simulink library "STMM"  (R2024a)
settings: Solver=VariableStepAuto  StartTime=0.0  StopTime=10.0  RelTol=1e-3
undefined symbols (not defined in the file or in its folder): raptor_xcp_function, StateCAN
libraries: Utilities x260, Raptor_lib x68, simulink x2
(part 2 of 3)

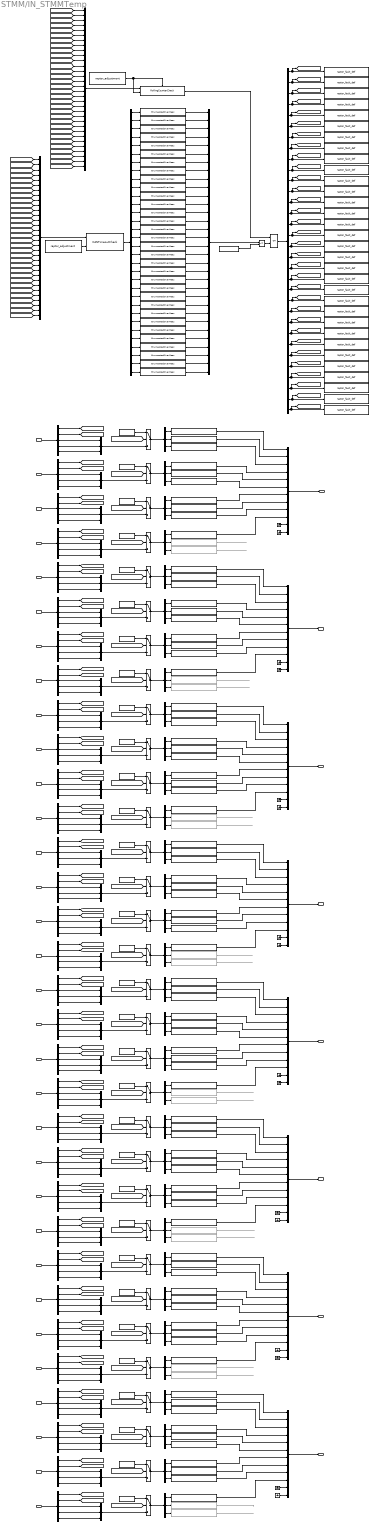
== system STMM/IN_STMMTemp ==
  IO_CAN2_300_Bus : Inport
  IO_CAN2_301_Bus : Inport  Port=2
  IO_CAN2_302_Bus : Inport  Port=3
  IO_CAN2_303_Bus : Inport  Port=4
  IO_CAN2_304_Bus : Inport  Port=5
  IO_CAN2_305_Bus : Inport  Port=6
  IO_CAN2_306_Bus : Inport  Port=7
  IO_CAN2_307_Bus : Inport  Port=8
  IO_CAN2_308_Bus : Inport  Port=9
  IO_CAN2_309_Bus : Inport  Port=10
  IO_CAN2_310_Bus : Inport  Port=11
  IO_CAN2_311_Bus : Inport  Port=12
  IO_CAN2_312_Bus : Inport  Port=13
  IO_CAN2_313_Bus : Inport  Port=14
  IO_CAN2_314_Bus : Inport  Port=15
  IO_CAN2_315_Bus : Inport  Port=16
  IO_CAN2_316_Bus : Inport  Port=17
  IO_CAN2_317_Bus : Inport  Port=18
  IO_CAN2_318_Bus : Inport  Port=19
  IO_CAN2_319_Bus : Inport  Port=20
  IO_CAN2_320_Bus : Inport  Port=21
  IO_CAN2_321_Bus : Inport  Port=22
  IO_CAN2_322_Bus : Inport  Port=23
  IO_CAN2_323_Bus : Inport  Port=24
  IO_CAN2_324_Bus : Inport  Port=25
  IO_CAN2_325_Bus : Inport  Port=26
  IO_CAN2_326_Bus : Inport  Port=27
  IO_CAN2_327_Bus : Inport  Port=28
  IO_CAN2_328_Bus : Inport  Port=29
  IO_CAN2_329_Bus : Inport  Port=30
  IO_CAN2_330_Bus : Inport  Port=31
  IO_CAN2_331_Bus : Inport  Port=32
  Bus Creator{,1..7} (8 alike) : BusCreator  Inputs=12
  Bus Selector : BusSelector  OutputSignals=Age,STMM_counterMsg300,STMM_segmentTemp100,STMM_segmentTemp101,STMM_segmentTemp102
  Bus Selector1 : BusSelector  OutputSignals=Age,STMM_counterMsg301,STMM_segmentTemp103,STMM_segmentTemp104,STMM_segmentTemp105
  Bus Selector10 : BusSelector  OutputSignals=Age,STMM_counterMsg310,STMM_segmentTemp306,STMM_segmentTemp307,STMM_segmentTemp308
  Bus Selector11 : BusSelector  OutputSignals=Age,STMM_counterMsg311,STMM_segmentTemp309,STMM_segmentTemp310,STMM_segmentTemp311
  Bus Selector12 : BusSelector  OutputSignals=Age,STMM_counterMsg312,STMM_segmentTemp400,STMM_segmentTemp401,STMM_segmentTemp402
  Bus Selector13 : BusSelector  OutputSignals=Age,STMM_counterMsg313,STMM_segmentTemp403,STMM_segmentTemp404,STMM_segmentTemp405
  Bus Selector14 : BusSelector  OutputSignals=Age,STMM_counterMsg314,STMM_segmentTemp406,STMM_segmentTemp407,STMM_segmentTemp408
  Bus Selector15 : BusSelector  OutputSignals=Age,STMM_counterMsg315,STMM_segmentTemp409,STMM_segmentTemp410,STMM_segmentTemp411
  Bus Selector16 : BusSelector  OutputSignals=Age,STMM_counterMsg316,STMM_segmentTemp500,STMM_segmentTemp501,STMM_segmentTemp502
  Bus Selector17 : BusSelector  OutputSignals=Age,STMM_counterMsg317,STMM_segmentTemp503,STMM_segmentTemp504,STMM_segmentTemp505
  Bus Selector18 : BusSelector  OutputSignals=Age,STMM_counterMsg318,STMM_segmentTemp506,STMM_segmentTemp507,STMM_segmentTemp508
  Bus Selector19 : BusSelector  OutputSignals=Age,STMM_counterMsg319,STMM_segmentTemp509,STMM_segmentTemp510,STMM_segmentTemp511
  Bus Selector2 : BusSelector  OutputSignals=Age,STMM_counterMsg302,STMM_segmentTemp106,STMM_segmentTemp107,STMM_segmentTemp108
  Bus Selector20 : BusSelector  OutputSignals=Age,STMM_counterMsg320,STMM_segmentTemp600,STMM_segmentTemp601,STMM_segmentTemp602
  Bus Selector21 : BusSelector  OutputSignals=Age,STMM_counterMsg321,STMM_segmentTemp603,STMM_segmentTemp604,STMM_segmentTemp605
  Bus Selector22 : BusSelector  OutputSignals=Age,STMM_counterMsg322,STMM_segmentTemp606,STMM_segmentTemp607,STMM_segmentTemp608
  Bus Selector23 : BusSelector  OutputSignals=Age,STMM_counterMsg323,STMM_segmentTemp609,STMM_segmentTemp610,STMM_segmentTemp611
  Bus Selector24 : BusSelector  OutputSignals=Age,STMM_counterMsg324,STMM_segmentTemp700,STMM_segmentTemp701,STMM_segmentTemp702
  Bus Selector25 : BusSelector  OutputSignals=Age,STMM_counterMsg325,STMM_segmentTemp703,STMM_segmentTemp704,STMM_segmentTemp705
  Bus Selector26 : BusSelector  OutputSignals=Age,STMM_counterMsg326,STMM_segmentTemp706,STMM_segmentTemp707,STMM_segmentTemp708
  Bus Selector27 : BusSelector  OutputSignals=Age,STMM_counterMsg327,STMM_segmentTemp709,STMM_segmentTemp710,STMM_segmentTemp711
  Bus Selector28 : BusSelector  OutputSignals=Age,STMM_counterMsg328,STMM_segmentTemp800,STMM_segmentTemp801,STMM_segmentTemp802
  Bus Selector29 : BusSelector  OutputSignals=Age,STMM_counterMsg329,STMM_segmentTemp803,STMM_segmentTemp804,STMM_segmentTemp805
  Bus Selector3 : BusSelector  OutputSignals=Age,STMM_counterMsg303,STMM_segmentTemp109,STMM_segmentTemp110,STMM_segmentTemp111
  Bus Selector30 : BusSelector  OutputSignals=Age,STMM_counterMsg330,STMM_segmentTemp806,STMM_segmentTemp807,STMM_segmentTemp808
  Bus Selector31 : BusSelector  OutputSignals=Age,STMM_counterMsg331,STMM_segmentTemp809,STMM_segmentTemp810,STMM_segmentTemp811
  Bus Selector4 : BusSelector  OutputSignals=Age,STMM_counterMsg304,STMM_segmentTemp200,STMM_segmentTemp201,STMM_segmentTemp202
  Bus Selector5 : BusSelector  OutputSignals=Age,STMM_counterMsg305,STMM_segmentTemp203,STMM_segmentTemp204,STMM_segmentTemp205
  Bus Selector6 : BusSelector  OutputSignals=Age,STMM_counterMsg306,STMM_segmentTemp206,STMM_segmentTemp207,STMM_segmentTemp208
  Bus Selector7 : BusSelector  OutputSignals=Age,STMM_counterMsg307,STMM_segmentTemp209,STMM_segmentTemp210,STMM_segmentTemp211
  Bus Selector8 : BusSelector  OutputSignals=Age,STMM_counterMsg308,STMM_segmentTemp300,STMM_segmentTemp301,STMM_segmentTemp302
  Bus Selector9 : BusSelector  OutputSignals=Age,STMM_counterMsg309,STMM_segmentTemp303,STMM_segmentTemp304,STMM_segmentTemp305
  CANTimeoutCheck : Utilities/CANTimeoutCheck
  Constant{1..32} (32 alike) : Constant  Value=int16(32767)
  Demux : Demux  Outputs=32
  Demux1 : Demux  Outputs=32
  Demux{2..33} (32 alike) : Demux  Outputs=3
  Enumerated Constant : simulink/Sources/Enumerated Constant  OutDataTypeStr=Enum: StateCAN  Value=StateCAN.Normal  SampleTime=inf
  EnumeratedOverMeas1 : Utilities/EnumeratedOverMeas  sigName='IN_CAN2_300_Status_en'  enumName='StateCAN'
  EnumeratedOverMeas10 : Utilities/EnumeratedOverMeas  sigName='IN_CAN2_309_Status_en'  enumName='StateCAN'
  EnumeratedOverMeas11 : Utilities/EnumeratedOverMeas  sigName='IN_CAN2_310_Status_en'  enumName='StateCAN'
  EnumeratedOverMeas12 : Utilities/EnumeratedOverMeas  sigName='IN_CAN2_311_Status_en'  enumName='StateCAN'
  EnumeratedOverMeas13 : Utilities/EnumeratedOverMeas  sigName='IN_CAN2_312_Status_en'  enumName='StateCAN'
  EnumeratedOverMeas14 : Utilities/EnumeratedOverMeas  sigName='IN_CAN2_313_Status_en'  enumName='StateCAN'
  EnumeratedOverMeas15 : Utilities/EnumeratedOverMeas  sigName='IN_CAN2_314_Status_en'  enumName='StateCAN'
  EnumeratedOverMeas16 : Utilities/EnumeratedOverMeas  sigName='IN_CAN2_315_Status_en'  enumName='StateCAN'
  EnumeratedOverMeas17 : Utilities/EnumeratedOverMeas  sigName='IN_CAN2_316_Status_en'  enumName='StateCAN'
  EnumeratedOverMeas18 : Utilities/EnumeratedOverMeas  sigName='IN_CAN2_317_Status_en'  enumName='StateCAN'
  EnumeratedOverMeas19 : Utilities/EnumeratedOverMeas  sigName='IN_CAN2_318_Status_en'  enumName='StateCAN'
  EnumeratedOverMeas2 : Utilities/EnumeratedOverMeas  sigName='IN_CAN2_301_Status_en'  enumName='StateCAN'
  EnumeratedOverMeas20 : Utilities/EnumeratedOverMeas  sigName='IN_CAN2_319_Status_en'  enumName='StateCAN'
  EnumeratedOverMeas21 : Utilities/EnumeratedOverMeas  sigName='IN_CAN2_320_Status_en'  enumName='StateCAN'
  EnumeratedOverMeas22 : Utilities/EnumeratedOverMeas  sigName='IN_CAN2_321_Status_en'  enumName='StateCAN'
  EnumeratedOverMeas23 : Utilities/EnumeratedOverMeas  sigName='IN_CAN2_322_Status_en'  enumName='StateCAN'
  EnumeratedOverMeas24 : Utilities/EnumeratedOverMeas  sigName='IN_CAN2_323_Status_en'  enumName='StateCAN'
  EnumeratedOverMeas25 : Utilities/EnumeratedOverMeas  sigName='IN_CAN2_324_Status_en'  enumName='StateCAN'
  EnumeratedOverMeas26 : Utilities/EnumeratedOverMeas  sigName='IN_CAN2_325_Status_en'  enumName='StateCAN'
  EnumeratedOverMeas27 : Utilities/EnumeratedOverMeas  sigName='IN_CAN2_326_Status_en'  enumName='StateCAN'
  EnumeratedOverMeas28 : Utilities/EnumeratedOverMeas  sigName='IN_CAN2_327_Status_en'  enumName='StateCAN'
  EnumeratedOverMeas29 : Utilities/EnumeratedOverMeas  sigName='IN_CAN2_328_Status_en'  enumName='StateCAN'
  EnumeratedOverMeas3 : Utilities/EnumeratedOverMeas  sigName='IN_CAN2_302_Status_en'  enumName='StateCAN'
  EnumeratedOverMeas30 : Utilities/EnumeratedOverMeas  sigName='IN_CAN2_329_Status_en'  enumName='StateCAN'
  EnumeratedOverMeas31 : Utilities/EnumeratedOverMeas  sigName='IN_CAN2_330_Status_en'  enumName='StateCAN'
  EnumeratedOverMeas32 : Utilities/EnumeratedOverMeas  sigName='IN_CAN2_331_Status_en'  enumName='StateCAN'
  EnumeratedOverMeas4 : Utilities/EnumeratedOverMeas  sigName='IN_CAN2_303_Status_en'  enumName='StateCAN'
  EnumeratedOverMeas5 : Utilities/EnumeratedOverMeas  sigName='IN_CAN2_304_Status_en'  enumName='StateCAN'
  EnumeratedOverMeas6 : Utilities/EnumeratedOverMeas  sigName='IN_CAN2_305_Status_en'  enumName='StateCAN'
  EnumeratedOverMeas7 : Utilities/EnumeratedOverMeas  sigName='IN_CAN2_306_Status_en'  enumName='StateCAN'
  EnumeratedOverMeas8 : Utilities/EnumeratedOverMeas  sigName='IN_CAN2_307_Status_en'  enumName='StateCAN'
  EnumeratedOverMeas9 : Utilities/EnumeratedOverMeas  sigName='IN_CAN2_308_Status_en'  enumName='StateCAN'
  Equal : RelationalOperator  Operator=~=  OutDataTypeStr=boolean  RndMeth=Simplest  InputSameDT=off
  Ground{,1..15} (16 alike) : Ground
  Mux{,1..31} (32 alike) : Mux  Inputs=3
  Mux32 : Mux  Inputs=32
  Mux33 : Mux  Inputs=32
  Mux34 : Mux  Inputs=32
  OR : Logic  Operator=OR  AllPortsSameDT=off  OutDataTypeStr=boolean
  OverMeas : Utilities/OverMeas  sigName='IN_SegmentTemp100_degC'  minimum=-inf  maximum=inf
  OverMeas1 : Utilities/OverMeas  sigName='IN_SegmentTemp101_degC'  minimum=-inf  maximum=inf
  OverMeas10 : Utilities/OverMeas  Commented=on  sigName='IN_SegmentTemp110_degC'  minimum=-inf  maximum=inf
  OverMeas11 : Utilities/OverMeas  Commented=on  sigName='IN_SegmentTemp111_degC'  minimum=-inf  maximum=inf
  OverMeas12 : Utilities/OverMeas  sigName='IN_SegmentTemp200_degC'  minimum=-inf  maximum=inf
  OverMeas13 : Utilities/OverMeas  sigName='IN_SegmentTemp201_degC'  minimum=-inf  maximum=inf
  OverMeas14 : Utilities/OverMeas  Commented=on  sigName='IN_SegmentTemp210_degC'  minimum=-inf  maximum=inf
  OverMeas15 : Utilities/OverMeas  Commented=on  sigName='IN_SegmentTemp211_degC'  minimum=-inf  maximum=inf
  OverMeas16 : Utilities/OverMeas  sigName='IN_SegmentTemp202_degC'  minimum=-inf  maximum=inf
  OverMeas17 : Utilities/OverMeas  sigName='IN_SegmentTemp203_degC'  minimum=-inf  maximum=inf
  OverMeas18 : Utilities/OverMeas  sigName='IN_SegmentTemp204_degC'  minimum=-inf  maximum=inf
  OverMeas19 : Utilities/OverMeas  sigName='IN_SegmentTemp205_degC'  minimum=-inf  maximum=inf
  OverMeas2 : Utilities/OverMeas  sigName='IN_SegmentTemp102_degC'  minimum=-inf  maximum=inf
  OverMeas20 : Utilities/OverMeas  sigName='IN_SegmentTemp206_degC'  minimum=-inf  maximum=inf
  OverMeas21 : Utilities/OverMeas  sigName='IN_SegmentTemp207_degC'  minimum=-inf  maximum=inf
  OverMeas22 : Utilities/OverMeas  sigName='IN_SegmentTemp208_degC'  minimum=-inf  maximum=inf
  OverMeas23 : Utilities/OverMeas  sigName='IN_SegmentTemp209_degC'  minimum=-inf  maximum=inf
  OverMeas24 : Utilities/OverMeas  sigName='IN_SegmentTemp300_degC'  minimum=-inf  maximum=inf
  OverMeas25 : Utilities/OverMeas  sigName='IN_SegmentTemp301_degC'  minimum=-inf  maximum=inf
  OverMeas26 : Utilities/OverMeas  Commented=on  sigName='IN_SegmentTemp310_degC'  minimum=-inf  maximum=inf
  OverMeas27 : Utilities/OverMeas  Commented=on  sigName='IN_SegmentTemp311_degC'  minimum=-inf  maximum=inf
  OverMeas28 : Utilities/OverMeas  sigName='IN_SegmentTemp302_degC'  minimum=-inf  maximum=inf
  OverMeas29 : Utilities/OverMeas  sigName='IN_SegmentTemp303_degC'  minimum=-inf  maximum=inf
  OverMeas3 : Utilities/OverMeas  sigName='IN_SegmentTemp103_degC'  minimum=-inf  maximum=inf
  OverMeas30 : Utilities/OverMeas  sigName='IN_SegmentTemp304_degC'  minimum=-inf  maximum=inf
  OverMeas31 : Utilities/OverMeas  sigName='IN_SegmentTemp305_degC'  minimum=-inf  maximum=inf
  OverMeas32 : Utilities/OverMeas  sigName='IN_SegmentTemp306_degC'  minimum=-inf  maximum=inf
  OverMeas33 : Utilities/OverMeas  sigName='IN_SegmentTemp307_degC'  minimum=-inf  maximum=inf
  OverMeas34 : Utilities/OverMeas  sigName='IN_SegmentTemp308_degC'  minimum=-inf  maximum=inf
  OverMeas35 : Utilities/OverMeas  sigName='IN_SegmentTemp309_degC'  minimum=-inf  maximum=inf
  OverMeas36 : Utilities/OverMeas  sigName='IN_SegmentTemp400_degC'  minimum=-inf  maximum=inf
  OverMeas37 : Utilities/OverMeas  sigName='IN_SegmentTemp401_degC'  minimum=-inf  maximum=inf
  OverMeas38 : Utilities/OverMeas  Commented=on  sigName='IN_SegmentTemp410_degC'  minimum=-inf  maximum=inf
  OverMeas39 : Utilities/OverMeas  Commented=on  sigName='IN_SegmentTemp411_degC'  minimum=-inf  maximum=inf
  OverMeas4 : Utilities/OverMeas  sigName='IN_SegmentTemp104_degC'  minimum=-inf  maximum=inf
  OverMeas40 : Utilities/OverMeas  sigName='IN_SegmentTemp402_degC'  minimum=-inf  maximum=inf
  OverMeas41 : Utilities/OverMeas  sigName='IN_SegmentTemp403_degC'  minimum=-inf  maximum=inf
  OverMeas42 : Utilities/OverMeas  sigName='IN_SegmentTemp404_degC'  minimum=-inf  maximum=inf
  OverMeas43 : Utilities/OverMeas  sigName='IN_SegmentTemp405_degC'  minimum=-inf  maximum=inf
  OverMeas44 : Utilities/OverMeas  sigName='IN_SegmentTemp406_degC'  minimum=-inf  maximum=inf
  OverMeas45 : Utilities/OverMeas  sigName='IN_SegmentTemp407_degC'  minimum=-inf  maximum=inf
  OverMeas46 : Utilities/OverMeas  sigName='IN_SegmentTemp408_degC'  minimum=-inf  maximum=inf
  OverMeas47 : Utilities/OverMeas  sigName='IN_SegmentTemp409_degC'  minimum=-inf  maximum=inf
  OverMeas48 : Utilities/OverMeas  sigName='IN_SegmentTemp500_degC'  minimum=-inf  maximum=inf
  OverMeas49 : Utilities/OverMeas  sigName='IN_SegmentTemp501_degC'  minimum=-inf  maximum=inf
  OverMeas5 : Utilities/OverMeas  sigName='IN_SegmentTemp105_degC'  minimum=-inf  maximum=inf
  OverMeas50 : Utilities/OverMeas  Commented=on  sigName='IN_SegmentTemp510_degC'  minimum=-inf  maximum=inf
  OverMeas51 : Utilities/OverMeas  Commented=on  sigName='IN_SegmentTemp511_degC'  minimum=-inf  maximum=inf
  OverMeas52 : Utilities/OverMeas  sigName='IN_SegmentTemp502_degC'  minimum=-inf  maximum=inf
  OverMeas53 : Utilities/OverMeas  sigName='IN_SegmentTemp503_degC'  minimum=-inf  maximum=inf
  OverMeas54 : Utilities/OverMeas  sigName='IN_SegmentTemp504_degC'  minimum=-inf  maximum=inf
  OverMeas55 : Utilities/OverMeas  sigName='IN_SegmentTemp505_degC'  minimum=-inf  maximum=inf
  OverMeas56 : Utilities/OverMeas  sigName='IN_SegmentTemp506_degC'  minimum=-inf  maximum=inf
  OverMeas57 : Utilities/OverMeas  sigName='IN_SegmentTemp507_degC'  minimum=-inf  maximum=inf
  OverMeas58 : Utilities/OverMeas  sigName='IN_SegmentTemp508_degC'  minimum=-inf  maximum=inf
  OverMeas59 : Utilities/OverMeas  sigName='IN_SegmentTemp509_degC'  minimum=-inf  maximum=inf
  OverMeas6 : Utilities/OverMeas  sigName='IN_SegmentTemp106_degC'  minimum=-inf  maximum=inf
  OverMeas60 : Utilities/OverMeas  sigName='IN_SegmentTemp600_degC'  minimum=-inf  maximum=inf
  OverMeas61 : Utilities/OverMeas  sigName='IN_SegmentTemp601_degC'  minimum=-inf  maximum=inf
  OverMeas62 : Utilities/OverMeas  Commented=on  sigName='IN_SegmentTemp610_degC'  minimum=-inf  maximum=inf
  OverMeas63 : Utilities/OverMeas  Commented=on  sigName='IN_SegmentTemp611_degC'  minimum=-inf  maximum=inf
  OverMeas64 : Utilities/OverMeas  sigName='IN_SegmentTemp602_degC'  minimum=-inf  maximum=inf
  OverMeas65 : Utilities/OverMeas  sigName='IN_SegmentTemp603_degC'  minimum=-inf  maximum=inf
  OverMeas66 : Utilities/OverMeas  sigName='IN_SegmentTemp604_degC'  minimum=-inf  maximum=inf
  OverMeas67 : Utilities/OverMeas  sigName='IN_SegmentTemp605_degC'  minimum=-inf  maximum=inf
  OverMeas68 : Utilities/OverMeas  sigName='IN_SegmentTemp606_degC'  minimum=-inf  maximum=inf
  OverMeas69 : Utilities/OverMeas  sigName='IN_SegmentTemp607_degC'  minimum=-inf  maximum=inf
  OverMeas7 : Utilities/OverMeas  sigName='IN_SegmentTemp107_degC'  minimum=-inf  maximum=inf
  OverMeas70 : Utilities/OverMeas  sigName='IN_SegmentTemp608_degC'  minimum=-inf  maximum=inf
  OverMeas71 : Utilities/OverMeas  sigName='IN_SegmentTemp609_degC'  minimum=-inf  maximum=inf
  OverMeas72 : Utilities/OverMeas  sigName='IN_SegmentTemp700_degC'  minimum=-inf  maximum=inf
  OverMeas73 : Utilities/OverMeas  sigName='IN_SegmentTemp701_degC'  minimum=-inf  maximum=inf
  OverMeas74 : Utilities/OverMeas  Commented=on  sigName='IN_SegmentTemp710_degC'  minimum=-inf  maximum=inf
  OverMeas75 : Utilities/OverMeas  Commented=on  sigName='IN_SegmentTemp711_degC'  minimum=-inf  maximum=inf
  OverMeas76 : Utilities/OverMeas  sigName='IN_SegmentTemp702_degC'  minimum=-inf  maximum=inf
  OverMeas77 : Utilities/OverMeas  sigName='IN_SegmentTemp703_degC'  minimum=-inf  maximum=inf
  OverMeas78 : Utilities/OverMeas  sigName='IN_SegmentTemp704_degC'  minimum=-inf  maximum=inf
  OverMeas79 : Utilities/OverMeas  sigName='IN_SegmentTemp705_degC'  minimum=-inf  maximum=inf
  OverMeas8 : Utilities/OverMeas  sigName='IN_SegmentTemp108_degC'  minimum=-inf  maximum=inf
  OverMeas80 : Utilities/OverMeas  sigName='IN_SegmentTemp706_degC'  minimum=-inf  maximum=inf
  OverMeas81 : Utilities/OverMeas  sigName='IN_SegmentTemp707_degC'  minimum=-inf  maximum=inf
  OverMeas82 : Utilities/OverMeas  sigName='IN_SegmentTemp708_degC'  minimum=-inf  maximum=inf
  OverMeas83 : Utilities/OverMeas  sigName='IN_SegmentTemp709_degC'  minimum=-inf  maximum=inf
  OverMeas84 : Utilities/OverMeas  sigName='IN_SegmentTemp800_degC'  minimum=-inf  maximum=inf
  OverMeas85 : Utilities/OverMeas  sigName='IN_SegmentTemp801_degC'  minimum=-inf  maximum=inf
  OverMeas86 : Utilities/OverMeas  Commented=on  sigName='IN_SegmentTemp810_degC'  minimum=-inf  maximum=inf
  OverMeas87 : Utilities/OverMeas  Commented=on  sigName='IN_SegmentTemp811_degC'  minimum=-inf  maximum=inf
  OverMeas88 : Utilities/OverMeas  sigName='IN_SegmentTemp802_degC'  minimum=-inf  maximum=inf
  OverMeas89 : Utilities/OverMeas  sigName='IN_SegmentTemp803_degC'  minimum=-inf  maximum=inf
  OverMeas9 : Utilities/OverMeas  sigName='IN_SegmentTemp109_degC'  minimum=-inf  maximum=inf
  OverMeas90 : Utilities/OverMeas  sigName='IN_SegmentTemp804_degC'  minimum=-inf  maximum=inf
  OverMeas91 : Utilities/OverMeas  sigName='IN_SegmentTemp805_degC'  minimum=-inf  maximum=inf
  OverMeas92 : Utilities/OverMeas  sigName='IN_SegmentTemp806_degC'  minimum=-inf  maximum=inf
  OverMeas93 : Utilities/OverMeas  sigName='IN_SegmentTemp807_degC'  minimum=-inf  maximum=inf
  OverMeas94 : Utilities/OverMeas  sigName='IN_SegmentTemp808_degC'  minimum=-inf  maximum=inf
  OverMeas95 : Utilities/OverMeas  sigName='IN_SegmentTemp809_degC'  minimum=-inf  maximum=inf
  RollingCounterCheck : Utilities/RollingCounterCheck
  Switch{1..32} (32 alike) : Switch  Criteria=u2 ~= 0  SaturateOnIntegerOverflow=off  InputSameDT=off
  raptor_adjustment : Raptor_lib/Data Storage/raptor_adjustment  paramName='IN_STMMTempTOThresh_na'  nameSource=Parameter  initValue=200  dataType=uint32  storage=Calibration  calDispType=Number  calEnum={'False', 'True'}  calGain=1.0  calOffset=0.0  calMax=inf  calMin=-inf  calFormat='-1'  calUnit=''  calHelp=''  calAccess=1  calFunction=raptor_xcp_function(gcb)  calDispHeaders=off  calColHeaders={'Col1' 'Col2' 'Col3'}  calRowHeaders={'Row1' 'Row2' 'Row3'}
      settings: SourceProductName=Raptor
  raptor_adjustment1 : Raptor_lib/Data Storage/raptor_adjustment  paramName='IN_STMMTempRollingCounterEnable_bool'  nameSource=Parameter  initValue=1  dataType=boolean  storage=Calibration  calDispType=Number  calEnum={'False', 'True'}  calGain=1.0  calOffset=0.0  calMax=inf  calMin=-inf  calFormat='-1'  calUnit=''  calHelp=''  calAccess=1  calFunction=raptor_xcp_function(gcb)  calDispHeaders=off  calColHeaders={'Col1' 'Col2' 'Col3'}  calRowHeaders={'Row1' 'Row2' 'Row3'}
      settings: SourceProductName=Raptor
  raptor_fault_def : Raptor_lib/Faults/raptor_fault_def  faultName='IN_CAN2_300_Fault'  persist=on  sticky=off  emisRelated=off  singleTrip=off  clearMethod=Standard  xLimit=25  yLimit=50  calEnable=on  addDisable=off  calAccess=1  calFunction='System | FaultManager'
      settings: SourceProductName=Raptor
  raptor_fault_def1 : Raptor_lib/Faults/raptor_fault_def  faultName='IN_CAN2_301_Fault'  persist=on  sticky=off  emisRelated=off  singleTrip=off  clearMethod=Standard  xLimit=25  yLimit=50  calEnable=on  addDisable=off  calAccess=1  calFunction='System | FaultManager'
      settings: SourceProductName=Raptor
  raptor_fault_def10 : Raptor_lib/Faults/raptor_fault_def  faultName='IN_CAN2_310_Fault'  persist=on  sticky=off  emisRelated=off  singleTrip=off  clearMethod=Standard  xLimit=25  yLimit=50  calEnable=on  addDisable=off  calAccess=1  calFunction='System | FaultManager'
      settings: SourceProductName=Raptor
  raptor_fault_def11 : Raptor_lib/Faults/raptor_fault_def  faultName='IN_CAN2_311_Fault'  persist=on  sticky=off  emisRelated=off  singleTrip=off  clearMethod=Standard  xLimit=25  yLimit=50  calEnable=on  addDisable=off  calAccess=1  calFunction='System | FaultManager'
      settings: SourceProductName=Raptor
  raptor_fault_def12 : Raptor_lib/Faults/raptor_fault_def  faultName='IN_CAN2_312_Fault'  persist=on  sticky=off  emisRelated=off  singleTrip=off  clearMethod=Standard  xLimit=25  yLimit=50  calEnable=on  addDisable=off  calAccess=1  calFunction='System | FaultManager'
      settings: SourceProductName=Raptor
  raptor_fault_def13 : Raptor_lib/Faults/raptor_fault_def  faultName='IN_CAN2_313_Fault'  persist=on  sticky=off  emisRelated=off  singleTrip=off  clearMethod=Standard  xLimit=25  yLimit=50  calEnable=on  addDisable=off  calAccess=1  calFunction='System | FaultManager'
      settings: SourceProductName=Raptor
  raptor_fault_def14 : Raptor_lib/Faults/raptor_fault_def  faultName='IN_CAN2_314_Fault'  persist=on  sticky=off  emisRelated=off  singleTrip=off  clearMethod=Standard  xLimit=25  yLimit=50  calEnable=on  addDisable=off  calAccess=1  calFunction='System | FaultManager'
      settings: SourceProductName=Raptor
  raptor_fault_def15 : Raptor_lib/Faults/raptor_fault_def  faultName='IN_CAN2_315_Fault'  persist=on  sticky=off  emisRelated=off  singleTrip=off  clearMethod=Standard  xLimit=25  yLimit=50  calEnable=on  addDisable=off  calAccess=1  calFunction='System | FaultManager'
      settings: SourceProductName=Raptor
  raptor_fault_def16 : Raptor_lib/Faults/raptor_fault_def  faultName='IN_CAN2_316_Fault'  persist=on  sticky=off  emisRelated=off  singleTrip=off  clearMethod=Standard  xLimit=25  yLimit=50  calEnable=on  addDisable=off  calAccess=1  calFunction='System | FaultManager'
      settings: SourceProductName=Raptor
  raptor_fault_def17 : Raptor_lib/Faults/raptor_fault_def  faultName='IN_CAN2_317_Fault'  persist=on  sticky=off  emisRelated=off  singleTrip=off  clearMethod=Standard  xLimit=25  yLimit=50  calEnable=on  addDisable=off  calAccess=1  calFunction='System | FaultManager'
      settings: SourceProductName=Raptor
  raptor_fault_def18 : Raptor_lib/Faults/raptor_fault_def  faultName='IN_CAN2_318_Fault'  persist=on  sticky=off  emisRelated=off  singleTrip=off  clearMethod=Standard  xLimit=25  yLimit=50  calEnable=on  addDisable=off  calAccess=1  calFunction='System | FaultManager'
      settings: SourceProductName=Raptor
  raptor_fault_def19 : Raptor_lib/Faults/raptor_fault_def  faultName='IN_CAN2_319_Fault'  persist=on  sticky=off  emisRelated=off  singleTrip=off  clearMethod=Standard  xLimit=25  yLimit=50  calEnable=on  addDisable=off  calAccess=1  calFunction='System | FaultManager'
      settings: SourceProductName=Raptor
  raptor_fault_def2 : Raptor_lib/Faults/raptor_fault_def  faultName='IN_CAN2_302_Fault'  persist=on  sticky=off  emisRelated=off  singleTrip=off  clearMethod=Standard  xLimit=25  yLimit=50  calEnable=on  addDisable=off  calAccess=1  calFunction='System | FaultManager'
      settings: SourceProductName=Raptor
  raptor_fault_def20 : Raptor_lib/Faults/raptor_fault_def  faultName='IN_CAN2_320_Fault'  persist=on  sticky=off  emisRelated=off  singleTrip=off  clearMethod=Standard  xLimit=25  yLimit=50  calEnable=on  addDisable=off  calAccess=1  calFunction='System | FaultManager'
      settings: SourceProductName=Raptor
  raptor_fault_def21 : Raptor_lib/Faults/raptor_fault_def  faultName='IN_CAN2_321_Fault'  persist=on  sticky=off  emisRelated=off  singleTrip=off  clearMethod=Standard  xLimit=25  yLimit=50  calEnable=on  addDisable=off  calAccess=1  calFunction='System | FaultManager'
      settings: SourceProductName=Raptor
  raptor_fault_def22 : Raptor_lib/Faults/raptor_fault_def  faultName='IN_CAN2_322_Fault'  persist=on  sticky=off  emisRelated=off  singleTrip=off  clearMethod=Standard  xLimit=25  yLimit=50  calEnable=on  addDisable=off  calAccess=1  calFunction='System | FaultManager'
      settings: SourceProductName=Raptor
  raptor_fault_def23 : Raptor_lib/Faults/raptor_fault_def  faultName='IN_CAN2_323_Fault'  persist=on  sticky=off  emisRelated=off  singleTrip=off  clearMethod=Standard  xLimit=25  yLimit=50  calEnable=on  addDisable=off  calAccess=1  calFunction='System | FaultManager'
      settings: SourceProductName=Raptor
  raptor_fault_def24 : Raptor_lib/Faults/raptor_fault_def  faultName='IN_CAN2_324_Fault'  persist=on  sticky=off  emisRelated=off  singleTrip=off  clearMethod=Standard  xLimit=25  yLimit=50  calEnable=on  addDisable=off  calAccess=1  calFunction='System | FaultManager'
      settings: SourceProductName=Raptor
  raptor_fault_def25 : Raptor_lib/Faults/raptor_fault_def  faultName='IN_CAN2_325_Fault'  persist=on  sticky=off  emisRelated=off  singleTrip=off  clearMethod=Standard  xLimit=25  yLimit=50  calEnable=on  addDisable=off  calAccess=1  calFunction='System | FaultManager'
      settings: SourceProductName=Raptor
  raptor_fault_def26 : Raptor_lib/Faults/raptor_fault_def  faultName='IN_CAN2_326_Fault'  persist=on  sticky=off  emisRelated=off  singleTrip=off  clearMethod=Standard  xLimit=25  yLimit=50  calEnable=on  addDisable=off  calAccess=1  calFunction='System | FaultManager'
      settings: SourceProductName=Raptor
  raptor_fault_def27 : Raptor_lib/Faults/raptor_fault_def  faultName='IN_CAN2_327_Fault'  persist=on  sticky=off  emisRelated=off  singleTrip=off  clearMethod=Standard  xLimit=25  yLimit=50  calEnable=on  addDisable=off  calAccess=1  calFunction='System | FaultManager'
      settings: SourceProductName=Raptor
  raptor_fault_def28 : Raptor_lib/Faults/raptor_fault_def  faultName='IN_CAN2_328_Fault'  persist=on  sticky=off  emisRelated=off  singleTrip=off  clearMethod=Standard  xLimit=25  yLimit=50  calEnable=on  addDisable=off  calAccess=1  calFunction='System | FaultManager'
      settings: SourceProductName=Raptor
  raptor_fault_def29 : Raptor_lib/Faults/raptor_fault_def  faultName='IN_CAN2_329_Fault'  persist=on  sticky=off  emisRelated=off  singleTrip=off  clearMethod=Standard  xLimit=25  yLimit=50  calEnable=on  addDisable=off  calAccess=1  calFunction='System | FaultManager'
      settings: SourceProductName=Raptor
  raptor_fault_def3 : Raptor_lib/Faults/raptor_fault_def  faultName='IN_CAN2_303_Fault'  persist=on  sticky=off  emisRelated=off  singleTrip=off  clearMethod=Standard  xLimit=25  yLimit=50  calEnable=on  addDisable=off  calAccess=1  calFunction='System | FaultManager'
      settings: SourceProductName=Raptor
  raptor_fault_def30 : Raptor_lib/Faults/raptor_fault_def  faultName='IN_CAN2_330_Fault'  persist=on  sticky=off  emisRelated=off  singleTrip=off  clearMethod=Standard  xLimit=25  yLimit=50  calEnable=on  addDisable=off  calAccess=1  calFunction='System | FaultManager'
      settings: SourceProductName=Raptor
  raptor_fault_def31 : Raptor_lib/Faults/raptor_fault_def  faultName='IN_CAN2_331_Fault'  persist=on  sticky=off  emisRelated=off  singleTrip=off  clearMethod=Standard  xLimit=25  yLimit=50  calEnable=on  addDisable=off  calAccess=1  calFunction='System | FaultManager'
      settings: SourceProductName=Raptor
  raptor_fault_def4 : Raptor_lib/Faults/raptor_fault_def  faultName='IN_CAN2_304_Fault'  persist=on  sticky=off  emisRelated=off  singleTrip=off  clearMethod=Standard  xLimit=25  yLimit=50  calEnable=on  addDisable=off  calAccess=1  calFunction='System | FaultManager'
      settings: SourceProductName=Raptor
  raptor_fault_def5 : Raptor_lib/Faults/raptor_fault_def  faultName='IN_CAN2_305_Fault'  persist=on  sticky=off  emisRelated=off  singleTrip=off  clearMethod=Standard  xLimit=25  yLimit=50  calEnable=on  addDisable=off  calAccess=1  calFunction='System | FaultManager'
      settings: SourceProductName=Raptor
  raptor_fault_def6 : Raptor_lib/Faults/raptor_fault_def  faultName='IN_CAN2_306_Fault'  persist=on  sticky=off  emisRelated=off  singleTrip=off  clearMethod=Standard  xLimit=25  yLimit=50  calEnable=on  addDisable=off  calAccess=1  calFunction='System | FaultManager'
      settings: SourceProductName=Raptor
  raptor_fault_def7 : Raptor_lib/Faults/raptor_fault_def  faultName='IN_CAN2_307_Fault'  persist=on  sticky=off  emisRelated=off  singleTrip=off  clearMethod=Standard  xLimit=25  yLimit=50  calEnable=on  addDisable=off  calAccess=1  calFunction='System | FaultManager'
      settings: SourceProductName=Raptor
  raptor_fault_def8 : Raptor_lib/Faults/raptor_fault_def  faultName='IN_CAN2_308_Fault'  persist=on  sticky=off  emisRelated=off  singleTrip=off  clearMethod=Standard  xLimit=25  yLimit=50  calEnable=on  addDisable=off  calAccess=1  calFunction='System | FaultManager'
      settings: SourceProductName=Raptor
  raptor_fault_def9 : Raptor_lib/Faults/raptor_fault_def  faultName='IN_CAN2_309_Fault'  persist=on  sticky=off  emisRelated=off  singleTrip=off  clearMethod=Standard  xLimit=25  yLimit=50  calEnable=on  addDisable=off  calAccess=1  calFunction='System | FaultManager'
      settings: SourceProductName=Raptor
  IN_Segment1Temp_Bus : Outport
  IN_Segment2Temp_Bus : Outport  Port=2
  IN_Segment3Temp_Bus : Outport  Port=3
  IN_Segment4Temp_Bus : Outport  Port=4
  IN_Segment5Temp_Bus : Outport  Port=5
  IN_Segment6Temp_Bus : Outport  Port=6
  IN_Segment7Temp_Bus : Outport  Port=7
  IN_Segment8Temp_Bus : Outport  Port=8
  wires:
  Ground15/1 -> Bus Creator7/12
  Ground14/1 -> Bus Creator7/11
  Ground13/1 -> Bus Creator6/12
  Ground12/1 -> Bus Creator6/11
  Ground11/1 -> Bus Creator5/12
  Ground10/1 -> Bus Creator5/11
  Ground9/1 -> Bus Creator4/12
  Ground8/1 -> Bus Creator4/11
  Ground7/1 -> Bus Creator3/12
  Ground6/1 -> Bus Creator3/11
  Ground5/1 -> Bus Creator2/12
  Ground4/1 -> Bus Creator2/11
  Ground3/1 -> Bus Creator1/12
  Ground2/1 -> Bus Creator1/11
  Ground1/1 -> Bus Creator/12
  Ground/1 -> Bus Creator/11
  OverMeas90/1 -> Bus Creator7/5  "IN_SegmentTemp804_degC"
  Demux31/3 -> OverMeas91/1
  OverMeas92/1 -> Bus Creator7/7  "IN_SegmentTemp806_degC"
  OverMeas91/1 -> Bus Creator7/6  "IN_SegmentTemp805_degC"
  OverMeas87/1 -> ?  "IN_SegmentTemp811_degC"
  Demux33/3 -> OverMeas87/1
  Switch31/1 -> Demux32/1
  Switch29/1 -> Demux30/1
  Switch30/1 -> Demux31/1
  Switch32/1 -> Demux33/1
  OverMeas88/1 -> Bus Creator7/3  "IN_SegmentTemp802_degC"
  Bus Creator7/1 -> IN_Segment8Temp_Bus/1  "IN_Segment8Temp_Bus"
  Demux32/3 -> OverMeas94/1
  OverMeas93/1 -> Bus Creator7/8  "IN_SegmentTemp807_degC"
  Demux31/2 -> OverMeas90/1
  Demux33/2 -> OverMeas86/1
  OverMeas95/1 -> Bus Creator7/10  "IN_SegmentTemp809_degC"
  Demux32/2 -> OverMeas93/1
  OverMeas85/1 -> Bus Creator7/2  "IN_SegmentTemp801_degC"
  Demux32/1 -> OverMeas92/1
  OverMeas94/1 -> Bus Creator7/9  "IN_SegmentTemp808_degC"
  OverMeas86/1 -> ?  "IN_SegmentTemp810_degC"
  Demux30/1 -> OverMeas84/1
  Demux33/1 -> OverMeas95/1
  Demux30/2 -> OverMeas85/1
  OverMeas84/1 -> Bus Creator7/1  "IN_SegmentTemp800_degC"
  Demux30/3 -> OverMeas88/1
  Demux31/1 -> OverMeas89/1
  OverMeas89/1 -> Bus Creator7/4  "IN_SegmentTemp803_degC"
  Demux29/2 -> OverMeas74/1
  Bus Creator6/1 -> IN_Segment7Temp_Bus/1  "IN_Segment7Temp_Bus"
  Demux27/2 -> OverMeas78/1
  OverMeas81/1 -> Bus Creator6/8  "IN_SegmentTemp707_degC"
  Demux28/3 -> OverMeas82/1
  OverMeas76/1 -> Bus Creator6/3  "IN_SegmentTemp702_degC"
  Demux28/1 -> OverMeas80/1
  OverMeas73/1 -> Bus Creator6/2  "IN_SegmentTemp701_degC"
  OverMeas83/1 -> Bus Creator6/10  "IN_SegmentTemp709_degC"
  Demux28/2 -> OverMeas81/1
  OverMeas82/1 -> Bus Creator6/9  "IN_SegmentTemp708_degC"
  OverMeas77/1 -> Bus Creator6/4  "IN_SegmentTemp703_degC"
  Demux27/1 -> OverMeas77/1
  Demux26/3 -> OverMeas76/1
  Demux26/2 -> OverMeas73/1
  OverMeas72/1 -> Bus Creator6/1  "IN_SegmentTemp700_degC"
  Demux29/1 -> OverMeas83/1
  Demux26/1 -> OverMeas72/1
  OverMeas74/1 -> ?  "IN_SegmentTemp710_degC"
  Demux29/3 -> OverMeas75/1
  OverMeas79/1 -> Bus Creator6/6  "IN_SegmentTemp705_degC"
  OverMeas80/1 -> Bus Creator6/7  "IN_SegmentTemp706_degC"
  OverMeas78/1 -> Bus Creator6/5  "IN_SegmentTemp704_degC"
  Demux27/3 -> OverMeas79/1
  OverMeas75/1 -> ?  "IN_SegmentTemp711_degC"
  Switch25/1 -> Demux26/1
  Switch27/1 -> Demux28/1
  Switch28/1 -> Demux29/1
  Switch26/1 -> Demux27/1
  Demux24/1 -> OverMeas68/1
  Demux25/2 -> OverMeas62/1
  Demux24/3 -> OverMeas70/1
  OverMeas65/1 -> Bus Creator5/4  "IN_SegmentTemp603_degC"
  Demux24/2 -> OverMeas69/1
  OverMeas71/1 -> Bus Creator5/10  "IN_SegmentTemp609_degC"
  OverMeas64/1 -> Bus Creator5/3  "IN_SegmentTemp602_degC"
  Demux23/2 -> OverMeas66/1
  Bus Creator5/1 -> IN_Segment6Temp_Bus/1  "IN_Segment6Temp_Bus"
  OverMeas63/1 -> ?  "IN_SegmentTemp611_degC"
  OverMeas60/1 -> Bus Creator5/1  "IN_SegmentTemp600_degC"
  Demux22/1 -> OverMeas60/1
  OverMeas62/1 -> ?  "IN_SegmentTemp610_degC"
  Demux23/1 -> OverMeas65/1
  Demux25/1 -> OverMeas71/1
  Demux22/2 -> OverMeas61/1
  Demux22/3 -> OverMeas64/1
  OverMeas69/1 -> Bus Creator5/8  "IN_SegmentTemp607_degC"
  Switch23/1 -> Demux24/1
  Switch22/1 -> Demux23/1
  Switch21/1 -> Demux22/1
  Switch24/1 -> Demux25/1
  OverMeas67/1 -> Bus Creator5/6  "IN_SegmentTemp605_degC"
  Demux25/3 -> OverMeas63/1
  Demux23/3 -> OverMeas67/1
  OverMeas70/1 -> Bus Creator5/9  "IN_SegmentTemp608_degC"
  OverMeas61/1 -> Bus Creator5/2  "IN_SegmentTemp601_degC"
  OverMeas66/1 -> Bus Creator5/5  "IN_SegmentTemp604_degC"
  OverMeas68/1 -> Bus Creator5/7  "IN_SegmentTemp606_degC"
  Demux19/1 -> OverMeas53/1
  Switch19/1 -> Demux20/1
  Switch17/1 -> Demux18/1
  OverMeas59/1 -> Bus Creator4/10  "IN_SegmentTemp509_degC"
  Switch20/1 -> Demux21/1
  Switch18/1 -> Demux19/1
  OverMeas53/1 -> Bus Creator4/4  "IN_SegmentTemp503_degC"
  Demux18/2 -> OverMeas49/1
  Bus Creator4/1 -> IN_Segment5Temp_Bus/1  "IN_Segment5Temp_Bus"
  Demux21/2 -> OverMeas50/1
  OverMeas51/1 -> ?  "IN_SegmentTemp511_degC"
  OverMeas57/1 -> Bus Creator4/8  "IN_SegmentTemp507_degC"
  Demux18/3 -> OverMeas52/1
  OverMeas52/1 -> Bus Creator4/3  "IN_SegmentTemp502_degC"
  OverMeas50/1 -> ?  "IN_SegmentTemp510_degC"
  OverMeas48/1 -> Bus Creator4/1  "IN_SegmentTemp500_degC"
  Demux19/2 -> OverMeas54/1
  Demux20/2 -> OverMeas57/1
  Demux20/3 -> OverMeas58/1
  Demux21/1 -> OverMeas59/1
  OverMeas56/1 -> Bus Creator4/7  "IN_SegmentTemp506_degC"
  Demux20/1 -> OverMeas56/1
  OverMeas55/1 -> Bus Creator4/6  "IN_SegmentTemp505_degC"
  OverMeas49/1 -> Bus Creator4/2  "IN_SegmentTemp501_degC"
  OverMeas54/1 -> Bus Creator4/5  "IN_SegmentTemp504_degC"
  Demux19/3 -> OverMeas55/1
  OverMeas58/1 -> Bus Creator4/9  "IN_SegmentTemp508_degC"
  Demux21/3 -> OverMeas51/1
  Demux18/1 -> OverMeas48/1
  Demux17/2 -> OverMeas38/1
  Bus Creator3/1 -> IN_Segment4Temp_Bus/1  "IN_Segment4Temp_Bus"
  OverMeas41/1 -> Bus Creator3/4  "IN_SegmentTemp403_degC"
  Demux14/2 -> OverMeas37/1
  OverMeas47/1 -> Bus Creator3/10  "IN_SegmentTemp409_degC"
  OverMeas39/1 -> ?  "IN_SegmentTemp411_degC"
  Demux14/1 -> OverMeas36/1
  Demux17/3 -> OverMeas39/1
  Demux15/3 -> OverMeas43/1
  OverMeas46/1 -> Bus Creator3/9  "IN_SegmentTemp408_degC"
  OverMeas42/1 -> Bus Creator3/5  "IN_SegmentTemp404_degC"
  OverMeas37/1 -> Bus Creator3/2  "IN_SegmentTemp401_degC"
  OverMeas43/1 -> Bus Creator3/6  "IN_SegmentTemp405_degC"
  Demux16/1 -> OverMeas44/1
  OverMeas44/1 -> Bus Creator3/7  "IN_SegmentTemp406_degC"
  Demux17/1 -> OverMeas47/1
  OverMeas40/1 -> Bus Creator3/3  "IN_SegmentTemp402_degC"
  Demux15/1 -> OverMeas41/1
  Switch16/1 -> Demux17/1
  Switch15/1 -> Demux16/1
  Demux16/3 -> OverMeas46/1
  Switch13/1 -> Demux14/1
  Switch14/1 -> Demux15/1
  OverMeas38/1 -> ?  "IN_SegmentTemp410_degC"
  OverMeas36/1 -> Bus Creator3/1  "IN_SegmentTemp400_degC"
  Demux15/2 -> OverMeas42/1
  Demux16/2 -> OverMeas45/1
  Demux14/3 -> OverMeas40/1
  OverMeas45/1 -> Bus Creator3/8  "IN_SegmentTemp407_degC"
  OverMeas29/1 -> Bus Creator2/4  "IN_SegmentTemp303_degC"
  Demux13/2 -> OverMeas26/1
  Demux11/3 -> OverMeas31/1
  OverMeas30/1 -> Bus Creator2/5  "IN_SegmentTemp304_degC"
  OverMeas35/1 -> Bus Creator2/10  "IN_SegmentTemp309_degC"
  Demux10/1 -> OverMeas24/1
  Demux13/3 -> OverMeas27/1
  Switch9/1 -> Demux10/1
  OverMeas26/1 -> ?  "IN_SegmentTemp310_degC"
  Switch12/1 -> Demux13/1
  OverMeas24/1 -> Bus Creator2/1  "IN_SegmentTemp300_degC"
  OverMeas32/1 -> Bus Creator2/7  "IN_SegmentTemp306_degC"
  Demux13/1 -> OverMeas35/1
  Demux11/1 -> OverMeas29/1
  OverMeas28/1 -> Bus Creator2/3  "IN_SegmentTemp302_degC"
  Switch11/1 -> Demux12/1
  Switch10/1 -> Demux11/1
  OverMeas31/1 -> Bus Creator2/6  "IN_SegmentTemp305_degC"
  OverMeas33/1 -> Bus Creator2/8  "IN_SegmentTemp307_degC"
  Demux12/3 -> OverMeas34/1
  Demux12/2 -> OverMeas33/1
  Demux11/2 -> OverMeas30/1
  OverMeas27/1 -> ?  "IN_SegmentTemp311_degC"
  Demux10/3 -> OverMeas28/1
  Demux10/2 -> OverMeas25/1
  Bus Creator2/1 -> IN_Segment3Temp_Bus/1  "IN_Segment3Temp_Bus"
  Demux12/1 -> OverMeas32/1
  OverMeas34/1 -> Bus Creator2/9  "IN_SegmentTemp308_degC"
  OverMeas25/1 -> Bus Creator2/2  "IN_SegmentTemp301_degC"
  Demux9/2 -> OverMeas14/1
  OverMeas16/1 -> Bus Creator1/3  "IN_SegmentTemp202_degC"
  Demux7/3 -> OverMeas19/1
  OverMeas17/1 -> Bus Creator1/4  "IN_SegmentTemp203_degC"
  Demux8/1 -> OverMeas20/1
  OverMeas20/1 -> Bus Creator1/7  "IN_SegmentTemp206_degC"
  Demux9/3 -> OverMeas15/1
  Demux6/2 -> OverMeas13/1
  Demux7/1 -> OverMeas17/1
  Switch5/1 -> Demux7/1
  Demux6/3 -> OverMeas16/1
  OverMeas15/1 -> ?  "IN_SegmentTemp211_degC"
  OverMeas23/1 -> Bus Creator1/10  "IN_SegmentTemp209_degC"
  Demux7/2 -> OverMeas18/1
  Switch7/1 -> Demux9/1
  Demux8/2 -> OverMeas21/1
  Demux8/3 -> OverMeas22/1
  OverMeas21/1 -> Bus Creator1/8  "IN_SegmentTemp207_degC"
  OverMeas19/1 -> Bus Creator1/6  "IN_SegmentTemp205_degC"
  OverMeas13/1 -> Bus Creator1/2  "IN_SegmentTemp201_degC"
  OverMeas22/1 -> Bus Creator1/9  "IN_SegmentTemp208_degC"
  OverMeas12/1 -> Bus Creator1/1  "IN_SegmentTemp200_degC"
  OverMeas18/1 -> Bus Creator1/5  "IN_SegmentTemp204_degC"
  Switch4/1 -> Demux6/1
  Demux6/1 -> OverMeas12/1
  Switch6/1 -> Demux8/1
  Bus Creator1/1 -> IN_Segment2Temp_Bus/1  "IN_Segment2Temp_Bus"
  OverMeas14/1 -> ?  "IN_SegmentTemp210_degC"
  Demux9/1 -> OverMeas23/1
  OverMeas11/1 -> ?  "IN_SegmentTemp111_degC"
  OverMeas10/1 -> ?  "IN_SegmentTemp110_degC"
  OverMeas9/1 -> Bus Creator/10  "IN_SegmentTemp109_degC"
  OverMeas8/1 -> Bus Creator/9  "IN_SegmentTemp108_degC"
  OverMeas7/1 -> Bus Creator/8  "IN_SegmentTemp107_degC"
  OverMeas6/1 -> Bus Creator/7  "IN_SegmentTemp106_degC"
  Demux5/3 -> OverMeas11/1
  Demux5/2 -> OverMeas10/1
  Demux5/1 -> OverMeas9/1
  Switch3/1 -> Demux5/1
  Demux4/3 -> OverMeas8/1
  Demux4/2 -> OverMeas7/1
  Demux4/1 -> OverMeas6/1
  Switch2/1 -> Demux4/1
  OverMeas5/1 -> Bus Creator/6  "IN_SegmentTemp105_degC"
  OverMeas4/1 -> Bus Creator/5  "IN_SegmentTemp104_degC"
  Demux3/3 -> OverMeas5/1
  Demux3/2 -> OverMeas4/1
  OverMeas3/1 -> Bus Creator/4  "IN_SegmentTemp103_degC"
  Demux3/1 -> OverMeas3/1
  Switch1/1 -> Demux3/1
  Bus Creator/1 -> IN_Segment1Temp_Bus/1  "IN_Segment1Temp_Bus"
  OverMeas2/1 -> Bus Creator/3  "IN_SegmentTemp102_degC"
  OverMeas1/1 -> Bus Creator/2  "IN_SegmentTemp101_degC"
  OverMeas/1 -> Bus Creator/1  "IN_SegmentTemp100_degC"
  Demux2/3 -> OverMeas2/1
  Demux2/2 -> OverMeas1/1
  Demux2/1 -> OverMeas/1
  Switch8/1 -> Demux2/1
  RollingCounterCheck/1 -> OR/1
  OR/1 -> Demux1/1
  raptor_adjustment1/1 -> RollingCounterCheck/Enable, RollingCounterCheck/2
  [IO_CAN2_331_cnt] -> Mux34/32
  [IO_CAN2_330_cnt] -> Mux34/31
  [IO_CAN2_329_cnt] -> Mux34/30
  [IO_CAN2_328_cnt] -> Mux34/29
  [IO_CAN2_327_cnt] -> Mux34/28
  [IO_CAN2_326_cnt] -> Mux34/27
  [IO_CAN2_325_cnt] -> Mux34/26
  [IO_CAN2_324_cnt] -> Mux34/25
  [IO_CAN2_323_cnt] -> Mux34/24
  [IO_CAN2_322_cnt] -> Mux34/23
  [IO_CAN2_321_cnt] -> Mux34/22
  [IO_CAN2_320_cnt] -> Mux34/21
  [IO_CAN2_319_cnt] -> Mux34/20
  [IO_CAN2_318_cnt] -> Mux34/19
  [IO_CAN2_317_cnt] -> Mux34/18
  [IO_CAN2_316_cnt] -> Mux34/17
  [IO_CAN2_315_cnt] -> Mux34/16
  [IO_CAN2_314_cnt] -> Mux34/15
  [IO_CAN2_313_cnt] -> Mux34/14
  [IO_CAN2_312_cnt] -> Mux34/13
  [IO_CAN2_311_cnt] -> Mux34/12
  [IO_CAN2_310_cnt] -> Mux34/11
  [IO_CAN2_309_cnt] -> Mux34/10
  [IO_CAN2_308_cnt] -> Mux34/9
  [IO_CAN2_307_cnt] -> Mux34/8
  [IO_CAN2_306_cnt] -> Mux34/7
  [IO_CAN2_305_cnt] -> Mux34/6
  [IO_CAN2_304_cnt] -> Mux34/5
  [IO_CAN2_303_cnt] -> Mux34/4
  [IO_CAN2_302_cnt] -> Mux34/3
  [IO_CAN2_301_cnt] -> Mux34/2
  [IO_CAN2_300_cnt] -> Mux34/1
  Mux34/1 -> RollingCounterCheck/1
  Mux31/1 -> Switch32/3
  Constant32/1 -> Switch32/1
  [IN_CAN2_331_Fault] -> Switch32/2
  Mux30/1 -> Switch31/3
  Constant31/1 -> Switch31/1
  [IN_CAN2_330_Fault] -> Switch31/2
  Mux29/1 -> Switch30/3
  Constant30/1 -> Switch30/1
  [IN_CAN2_329_Fault] -> Switch30/2
  Mux28/1 -> Switch29/3
  Constant29/1 -> Switch29/1
  [IN_CAN2_328_Fault] -> Switch29/2
  Constant28/1 -> Switch28/1
  [IN_CAN2_327_Fault] -> Switch28/2
  Mux27/1 -> Switch28/3
  Constant27/1 -> Switch27/1
  [IN_CAN2_326_Fault] -> Switch27/2
  Mux26/1 -> Switch27/3
  Constant26/1 -> Switch26/1
  [IN_CAN2_325_Fault] -> Switch26/2
  Mux25/1 -> Switch26/3
  Constant25/1 -> Switch25/1
  [IN_CAN2_324_Fault] -> Switch25/2
  Mux24/1 -> Switch25/3
  Constant24/1 -> Switch24/1
  [IN_CAN2_323_Fault] -> Switch24/2
  Mux23/1 -> Switch24/3
  Constant23/1 -> Switch23/1
  [IN_CAN2_322_Fault] -> Switch23/2
  Mux22/1 -> Switch23/3
  Constant22/1 -> Switch22/1
  [IN_CAN2_321_Fault] -> Switch22/2
  Mux21/1 -> Switch22/3
  Constant21/1 -> Switch21/1
  [IN_CAN2_320_Fault] -> Switch21/2
  Mux20/1 -> Switch21/3
  Constant20/1 -> Switch20/1
  [IN_CAN2_319_Fault] -> Switch20/2
  Mux19/1 -> Switch20/3
  Mux18/1 -> Switch19/3
  Constant19/1 -> Switch19/1
  [IN_CAN2_318_Fault] -> Switch19/2
  Mux17/1 -> Switch18/3
  Constant18/1 -> Switch18/1
  [IN_CAN2_317_Fault] -> Switch18/2
  Mux16/1 -> Switch17/3
  Constant17/1 -> Switch17/1
  [IN_CAN2_316_Fault] -> Switch17/2
  Mux15/1 -> Switch16/3
  Constant16/1 -> Switch16/1
  [IN_CAN2_315_Fault] -> Switch16/2
  Mux14/1 -> Switch15/3
  Constant15/1 -> Switch15/1
  [IN_CAN2_314_Fault] -> Switch15/2
  Mux13/1 -> Switch14/3
  Constant14/1 -> Switch14/1
  [IN_CAN2_313_Fault] -> Switch14/2
  Mux12/1 -> Switch13/3
  Constant13/1 -> Switch13/1
  [IN_CAN2_312_Fault] -> Switch13/2
  Mux11/1 -> Switch12/3
  Constant12/1 -> Switch12/1
  [IN_CAN2_311_Fault] -> Switch12/2
  Mux10/1 -> Switch11/3
  Constant11/1 -> Switch11/1
  [IN_CAN2_310_Fault] -> Switch11/2
  Mux9/1 -> Switch10/3
  Constant10/1 -> Switch10/1
  [IN_CAN2_309_Fault] -> Switch10/2
  Mux8/1 -> Switch9/3
  Constant9/1 -> Switch9/1
  [IN_CAN2_308_Fault] -> Switch9/2
  Mux7/1 -> Switch7/3
  Constant8/1 -> Switch7/1
  [IN_CAN2_307_Fault] -> Switch7/2
  Mux6/1 -> Switch6/3
  Constant7/1 -> Switch6/1
  [IN_CAN2_306_Fault] -> Switch6/2
  Mux5/1 -> Switch5/3
  Constant6/1 -> Switch5/1
  [IN_CAN2_305_Fault] -> Switch5/2
  Mux4/1 -> Switch4/3
  Constant5/1 -> Switch4/1
  [IN_CAN2_304_Fault] -> Switch4/2
  Mux3/1 -> Switch3/3
  Constant4/1 -> Switch3/1
  [IN_CAN2_303_Fault] -> Switch3/2
  Mux2/1 -> Switch2/3
  Constant3/1 -> Switch2/1
  [IN_CAN2_302_Fault] -> Switch2/2
  Mux1/1 -> Switch1/3
  Constant1/1 -> Switch1/1
  [IN_CAN2_301_Fault] -> Switch1/2
  Mux/1 -> Switch8/3
  [IN_CAN2_300_Fault] -> Switch8/2
  Constant2/1 -> Switch8/1
  Demux1/18 -> raptor_fault_def17/1, [IN_CAN2_317_Fault]
  Demux1/3 -> raptor_fault_def2/1, [IN_CAN2_302_Fault]
  Demux1/32 -> raptor_fault_def31/1, [IN_CAN2_331_Fault]
  Demux1/31 -> raptor_fault_def30/1, [IN_CAN2_330_Fault]
  Demux1/30 -> raptor_fault_def29/1, [IN_CAN2_329_Fault]
  Demux1/29 -> raptor_fault_def28/1, [IN_CAN2_328_Fault]
  Demux1/28 -> raptor_fault_def27/1, [IN_CAN2_327_Fault]
  Demux1/27 -> raptor_fault_def26/1, [IN_CAN2_326_Fault]
  Demux1/26 -> raptor_fault_def25/1, [IN_CAN2_325_Fault]
  Demux1/25 -> raptor_fault_def24/1, [IN_CAN2_324_Fault]
  Demux1/24 -> raptor_fault_def23/1, [IN_CAN2_323_Fault]
  Demux1/23 -> raptor_fault_def22/1, [IN_CAN2_322_Fault]
  Demux1/22 -> raptor_fault_def21/1, [IN_CAN2_321_Fault]
  Demux1/21 -> raptor_fault_def20/1, [IN_CAN2_320_Fault]
  Demux1/20 -> raptor_fault_def19/1, [IN_CAN2_319_Fault]
  Demux1/19 -> raptor_fault_def18/1, [IN_CAN2_318_Fault]
  Demux1/17 -> raptor_fault_def16/1, [IN_CAN2_316_Fault]
  Demux1/16 -> raptor_fault_def15/1, [IN_CAN2_315_Fault]
  Demux1/15 -> raptor_fault_def14/1, [IN_CAN2_314_Fault]
  Demux1/14 -> raptor_fault_def13/1, [IN_CAN2_313_Fault]
  Demux1/13 -> raptor_fault_def12/1, [IN_CAN2_312_Fault]
  Demux1/12 -> raptor_fault_def11/1, [IN_CAN2_311_Fault]
  Demux1/11 -> raptor_fault_def10/1, [IN_CAN2_310_Fault]
  Demux1/10 -> raptor_fault_def9/1, [IN_CAN2_309_Fault]
  Demux1/9 -> raptor_fault_def8/1, [IN_CAN2_308_Fault]
  Demux1/8 -> raptor_fault_def7/1, [IN_CAN2_307_Fault]
  Demux1/7 -> raptor_fault_def6/1, [IN_CAN2_306_Fault]
  Demux1/6 -> raptor_fault_def5/1, [IN_CAN2_305_Fault]
  Demux1/5 -> raptor_fault_def4/1, [IN_CAN2_304_Fault]
  Demux1/4 -> raptor_fault_def3/1, [IN_CAN2_303_Fault]
  Demux1/2 -> [IN_CAN2_301_Fault], raptor_fault_def1/1
  Demux1/1 -> [IN_CAN2_300_Fault], raptor_fault_def/1
  Equal/1 -> OR/2
  EnumeratedOverMeas32/1 -> Mux33/32  "IN_CAN2_331_Status_en"
  EnumeratedOverMeas31/1 -> Mux33/31  "IN_CAN2_330_Status_en"
  EnumeratedOverMeas30/1 -> Mux33/30  "IN_CAN2_329_Status_en"
  EnumeratedOverMeas29/1 -> Mux33/29  "IN_CAN2_328_Status_en"
  EnumeratedOverMeas28/1 -> Mux33/28  "IN_CAN2_327_Status_en"
  EnumeratedOverMeas27/1 -> Mux33/27  "IN_CAN2_326_Status_en"
  EnumeratedOverMeas26/1 -> Mux33/26  "IN_CAN2_325_Status_en"
  EnumeratedOverMeas25/1 -> Mux33/25  "IN_CAN2_324_Status_en"
  EnumeratedOverMeas24/1 -> Mux33/24  "IN_CAN2_323_Status_en"
  EnumeratedOverMeas23/1 -> Mux33/23  "IN_CAN2_322_Status_en"
  EnumeratedOverMeas22/1 -> Mux33/22  "IN_CAN2_321_Status_en"
  EnumeratedOverMeas21/1 -> Mux33/21  "IN_CAN2_320_Status_en"
  EnumeratedOverMeas20/1 -> Mux33/20  "IN_CAN2_319_Status_en"
  EnumeratedOverMeas19/1 -> Mux33/19  "IN_CAN2_318_Status_en"
  EnumeratedOverMeas18/1 -> Mux33/18  "IN_CAN2_317_Status_en"
  EnumeratedOverMeas17/1 -> Mux33/17  "IN_CAN2_316_Status_en"
  EnumeratedOverMeas16/1 -> Mux33/16  "IN_CAN2_315_Status_en"
  EnumeratedOverMeas15/1 -> Mux33/15  "IN_CAN2_314_Status_en"
  EnumeratedOverMeas14/1 -> Mux33/14  "IN_CAN2_313_Status_en"
  EnumeratedOverMeas13/1 -> Mux33/13  "IN_CAN2_312_Status_en"
  EnumeratedOverMeas12/1 -> Mux33/12  "IN_CAN2_311_Status_en"
  Demux/32 -> EnumeratedOverMeas32/1
  Demux/31 -> EnumeratedOverMeas31/1
  Demux/30 -> EnumeratedOverMeas30/1
  Demux/29 -> EnumeratedOverMeas29/1
  Demux/28 -> EnumeratedOverMeas28/1
  Demux/27 -> EnumeratedOverMeas27/1
  Demux/26 -> EnumeratedOverMeas26/1
  Demux/25 -> EnumeratedOverMeas25/1
  Demux/24 -> EnumeratedOverMeas24/1
  Demux/23 -> EnumeratedOverMeas23/1
  Demux/22 -> EnumeratedOverMeas22/1
  Demux/21 -> EnumeratedOverMeas21/1
  Demux/20 -> EnumeratedOverMeas20/1
  Demux/19 -> EnumeratedOverMeas19/1
  Demux/18 -> EnumeratedOverMeas18/1
  Demux/17 -> EnumeratedOverMeas17/1
  Demux/16 -> EnumeratedOverMeas16/1
  Demux/15 -> EnumeratedOverMeas15/1
  Demux/14 -> EnumeratedOverMeas14/1
  Demux/13 -> EnumeratedOverMeas13/1
  Demux/12 -> EnumeratedOverMeas12/1
  EnumeratedOverMeas11/1 -> Mux33/11  "IN_CAN2_310_Status_en"
  EnumeratedOverMeas10/1 -> Mux33/10  "IN_CAN2_309_Status_en"
  EnumeratedOverMeas9/1 -> Mux33/9  "IN_CAN2_308_Status_en"
  EnumeratedOverMeas8/1 -> Mux33/8  "IN_CAN2_307_Status_en"
  EnumeratedOverMeas7/1 -> Mux33/7  "IN_CAN2_306_Status_en"
  EnumeratedOverMeas6/1 -> Mux33/6  "IN_CAN2_305_Status_en"
  EnumeratedOverMeas5/1 -> Mux33/5  "IN_CAN2_304_Status_en"
  EnumeratedOverMeas4/1 -> Mux33/4  "IN_CAN2_303_Status_en"
  EnumeratedOverMeas3/1 -> Mux33/3  "IN_CAN2_302_Status_en"
  Demux/11 -> EnumeratedOverMeas11/1
  Demux/10 -> EnumeratedOverMeas10/1
  Demux/9 -> EnumeratedOverMeas9/1
  Demux/8 -> EnumeratedOverMeas8/1
  Demux/7 -> EnumeratedOverMeas7/1
  Demux/6 -> EnumeratedOverMeas6/1
  Demux/5 -> EnumeratedOverMeas5/1
  Demux/4 -> EnumeratedOverMeas4/1
  Demux/3 -> EnumeratedOverMeas3/1
  EnumeratedOverMeas2/1 -> Mux33/2  "IN_CAN2_301_Status_en"
  EnumeratedOverMeas1/1 -> Mux33/1  "IN_CAN2_300_Status_en"
  Demux/2 -> EnumeratedOverMeas2/1
  Demux/1 -> EnumeratedOverMeas1/1
  raptor_adjustment/1 -> CANTimeoutCheck/2
  Enumerated Constant/1 -> Equal/2
  Mux32/1 -> CANTimeoutCheck/1
  Mux33/1 -> Equal/1
  CANTimeoutCheck/1 -> Demux/1
  [IO_CAN2_331_Age] -> Mux32/32
  [IO_CAN2_330_Age] -> Mux32/31
  [IO_CAN2_329_Age] -> Mux32/30
  [IO_CAN2_328_Age] -> Mux32/29
  [IO_CAN2_327_Age] -> Mux32/28
  [IO_CAN2_326_Age] -> Mux32/27
  [IO_CAN2_325_Age] -> Mux32/26
  [IO_CAN2_324_Age] -> Mux32/25
  [IO_CAN2_323_Age] -> Mux32/24
  [IO_CAN2_322_Age] -> Mux32/23
  [IO_CAN2_321_Age] -> Mux32/22
  [IO_CAN2_320_Age] -> Mux32/21
  [IO_CAN2_319_Age] -> Mux32/20
  [IO_CAN2_318_Age] -> Mux32/19
  [IO_CAN2_317_Age] -> Mux32/18
  [IO_CAN2_316_Age] -> Mux32/17
  [IO_CAN2_315_Age] -> Mux32/16
  [IO_CAN2_314_Age] -> Mux32/15
  [IO_CAN2_313_Age] -> Mux32/14
  [IO_CAN2_312_Age] -> Mux32/13
  [IO_CAN2_311_Age] -> Mux32/12
  [IO_CAN2_310_Age] -> Mux32/11
  [IO_CAN2_309_Age] -> Mux32/10
  [IO_CAN2_308_Age] -> Mux32/9
  [IO_CAN2_307_Age] -> Mux32/8
  [IO_CAN2_306_Age] -> Mux32/7
  [IO_CAN2_305_Age] -> Mux32/6
  [IO_CAN2_304_Age] -> Mux32/5
  [IO_CAN2_303_Age] -> Mux32/4
  [IO_CAN2_302_Age] -> Mux32/3
  [IO_CAN2_301_Age] -> Mux32/2
  [IO_CAN2_300_Age] -> Mux32/1
  Bus Selector31/4 -> Mux31/2  "<STMM_segmentTemp810>"
  IO_CAN2_331_Bus/1 -> Bus Selector31/1
  Bus Selector31/5 -> Mux31/3  "<STMM_segmentTemp811>"
  Bus Selector31/3 -> Mux31/1  "<STMM_segmentTemp809>"
  Bus Selector31/2 -> [IO_CAN2_331_cnt]  "<STMM_counterMsg331>"
  Bus Selector31/1 -> [IO_CAN2_331_Age]  "<Age>"
  IO_CAN2_330_Bus/1 -> Bus Selector30/1
  Bus Selector30/3 -> Mux30/1  "<STMM_segmentTemp806>"
  Bus Selector30/4 -> Mux30/2  "<STMM_segmentTemp807>"
  Bus Selector30/2 -> [IO_CAN2_330_cnt]  "<STMM_counterMsg330>"
  Bus Selector30/5 -> Mux30/3  "<STMM_segmentTemp808>"
  Bus Selector30/1 -> [IO_CAN2_330_Age]  "<Age>"
  IO_CAN2_329_Bus/1 -> Bus Selector29/1
  Bus Selector29/1 -> [IO_CAN2_329_Age]  "<Age>"
  Bus Selector29/4 -> Mux29/2  "<STMM_segmentTemp804>"
  Bus Selector29/5 -> Mux29/3  "<STMM_segmentTemp805>"
  Bus Selector29/3 -> Mux29/1  "<STMM_segmentTemp803>"
  Bus Selector29/2 -> [IO_CAN2_329_cnt]  "<STMM_counterMsg329>"
  Bus Selector28/3 -> Mux28/1  "<STMM_segmentTemp800>"
  IO_CAN2_328_Bus/1 -> Bus Selector28/1
  Bus Selector28/2 -> [IO_CAN2_328_cnt]  "<STMM_counterMsg328>"
  Bus Selector28/4 -> Mux28/2  "<STMM_segmentTemp801>"
  Bus Selector28/1 -> [IO_CAN2_328_Age]  "<Age>"
  Bus Selector28/5 -> Mux28/3  "<STMM_segmentTemp802>"
  Bus Selector27/4 -> Mux27/2  "<STMM_segmentTemp710>"
  Bus Selector27/2 -> [IO_CAN2_327_cnt]  "<STMM_counterMsg327>"
  Bus Selector27/1 -> [IO_CAN2_327_Age]  "<Age>"
  IO_CAN2_327_Bus/1 -> Bus Selector27/1
  Bus Selector27/5 -> Mux27/3  "<STMM_segmentTemp711>"
  Bus Selector27/3 -> Mux27/1  "<STMM_segmentTemp709>"
  Bus Selector26/5 -> Mux26/3  "<STMM_segmentTemp708>"
  Bus Selector26/1 -> [IO_CAN2_326_Age]  "<Age>"
  IO_CAN2_326_Bus/1 -> Bus Selector26/1
  Bus Selector26/4 -> Mux26/2  "<STMM_segmentTemp707>"
  Bus Selector26/2 -> [IO_CAN2_326_cnt]  "<STMM_counterMsg326>"
  Bus Selector26/3 -> Mux26/1  "<STMM_segmentTemp706>"
  IO_CAN2_325_Bus/1 -> Bus Selector25/1
  Bus Selector25/5 -> Mux25/3  "<STMM_segmentTemp705>"
  Bus Selector25/3 -> Mux25/1  "<STMM_segmentTemp703>"
  Bus Selector25/1 -> [IO_CAN2_325_Age]  "<Age>"
  Bus Selector25/2 -> [IO_CAN2_325_cnt]  "<STMM_counterMsg325>"
  Bus Selector25/4 -> Mux25/2  "<STMM_segmentTemp704>"
  Bus Selector24/3 -> Mux24/1  "<STMM_segmentTemp700>"
  Bus Selector24/4 -> Mux24/2  "<STMM_segmentTemp701>"
  Bus Selector24/2 -> [IO_CAN2_324_cnt]  "<STMM_counterMsg324>"
  Bus Selector24/1 -> [IO_CAN2_324_Age]  "<Age>"
  IO_CAN2_324_Bus/1 -> Bus Selector24/1
  Bus Selector24/5 -> Mux24/3  "<STMM_segmentTemp702>"
  IO_CAN2_323_Bus/1 -> Bus Selector23/1
  Bus Selector23/2 -> [IO_CAN2_323_cnt]  "<STMM_counterMsg323>"
  Bus Selector23/4 -> Mux23/2  "<STMM_segmentTemp610>"
  Bus Selector23/3 -> Mux23/1  "<STMM_segmentTemp609>"
  Bus Selector23/5 -> Mux23/3  "<STMM_segmentTemp611>"
  Bus Selector23/1 -> [IO_CAN2_323_Age]  "<Age>"
  Bus Selector22/2 -> [IO_CAN2_322_cnt]  "<STMM_counterMsg322>"
  Bus Selector22/1 -> [IO_CAN2_322_Age]  "<Age>"
  Bus Selector22/5 -> Mux22/3  "<STMM_segmentTemp608>"
  Bus Selector22/4 -> Mux22/2  "<STMM_segmentTemp607>"
  Bus Selector22/3 -> Mux22/1  "<STMM_segmentTemp606>"
  IO_CAN2_322_Bus/1 -> Bus Selector22/1
  Bus Selector21/5 -> Mux21/3  "<STMM_segmentTemp605>"
  Bus Selector21/2 -> [IO_CAN2_321_cnt]  "<STMM_counterMsg321>"
  Bus Selector21/4 -> Mux21/2  "<STMM_segmentTemp604>"
  Bus Selector21/3 -> Mux21/1  "<STMM_segmentTemp603>"
  IO_CAN2_321_Bus/1 -> Bus Selector21/1
  Bus Selector21/1 -> [IO_CAN2_321_Age]  "<Age>"
  IO_CAN2_320_Bus/1 -> Bus Selector20/1
  Bus Selector20/2 -> [IO_CAN2_320_cnt]  "<STMM_counterMsg320>"
  Bus Selector20/4 -> Mux20/2  "<STMM_segmentTemp601>"
  Bus Selector20/5 -> Mux20/3  "<STMM_segmentTemp602>"
  Bus Selector20/3 -> Mux20/1  "<STMM_segmentTemp600>"
  Bus Selector20/1 -> [IO_CAN2_320_Age]  "<Age>"
  Bus Selector19/4 -> Mux19/2  "<STMM_segmentTemp510>"
  Bus Selector19/2 -> [IO_CAN2_319_cnt]  "<STMM_counterMsg319>"
  Bus Selector19/1 -> [IO_CAN2_319_Age]  "<Age>"
  Bus Selector19/5 -> Mux19/3  "<STMM_segmentTemp511>"
  Bus Selector19/3 -> Mux19/1  "<STMM_segmentTemp509>"
  IO_CAN2_319_Bus/1 -> Bus Selector19/1
  Bus Selector18/3 -> Mux18/1  "<STMM_segmentTemp506>"
  IO_CAN2_318_Bus/1 -> Bus Selector18/1
  Bus Selector18/1 -> [IO_CAN2_318_Age]  "<Age>"
  Bus Selector18/4 -> Mux18/2  "<STMM_segmentTemp507>"
  Bus Selector18/5 -> Mux18/3  "<STMM_segmentTemp508>"
  Bus Selector18/2 -> [IO_CAN2_318_cnt]  "<STMM_counterMsg318>"
  Bus Selector17/2 -> [IO_CAN2_317_cnt]  "<STMM_counterMsg317>"
  Bus Selector17/4 -> Mux17/2  "<STMM_segmentTemp504>"
  Bus Selector17/1 -> [IO_CAN2_317_Age]  "<Age>"
  Bus Selector17/5 -> Mux17/3  "<STMM_segmentTemp505>"
  IO_CAN2_317_Bus/1 -> Bus Selector17/1
  Bus Selector17/3 -> Mux17/1  "<STMM_segmentTemp503>"
  IO_CAN2_316_Bus/1 -> Bus Selector16/1
  Bus Selector16/3 -> Mux16/1  "<STMM_segmentTemp500>"
  Bus Selector16/5 -> Mux16/3  "<STMM_segmentTemp502>"
  Bus Selector16/2 -> [IO_CAN2_316_cnt]  "<STMM_counterMsg316>"
  Bus Selector16/1 -> [IO_CAN2_316_Age]  "<Age>"
  Bus Selector16/4 -> Mux16/2  "<STMM_segmentTemp501>"
  IO_CAN2_315_Bus/1 -> Bus Selector15/1
  Bus Selector15/2 -> [IO_CAN2_315_cnt]  "<STMM_counterMsg315>"
  Bus Selector15/3 -> Mux15/1  "<STMM_segmentTemp409>"
  Bus Selector15/1 -> [IO_CAN2_315_Age]  "<Age>"
  Bus Selector15/5 -> Mux15/3  "<STMM_segmentTemp411>"
  Bus Selector15/4 -> Mux15/2  "<STMM_segmentTemp410>"
  IO_CAN2_314_Bus/1 -> Bus Selector14/1
  Bus Selector14/4 -> Mux14/2  "<STMM_segmentTemp407>"
  Bus Selector14/3 -> Mux14/1  "<STMM_segmentTemp406>"
  Bus Selector14/5 -> Mux14/3  "<STMM_segmentTemp408>"
  Bus Selector14/1 -> [IO_CAN2_314_Age]  "<Age>"
  Bus Selector14/2 -> [IO_CAN2_314_cnt]  "<STMM_counterMsg314>"
  Bus Selector13/3 -> Mux13/1  "<STMM_segmentTemp403>"
  Bus Selector13/1 -> [IO_CAN2_313_Age]  "<Age>"
  Bus Selector13/2 -> [IO_CAN2_313_cnt]  "<STMM_counterMsg313>"
  Bus Selector13/5 -> Mux13/3  "<STMM_segmentTemp405>"
  Bus Selector13/4 -> Mux13/2  "<STMM_segmentTemp404>"
  IO_CAN2_313_Bus/1 -> Bus Selector13/1
  Bus Selector12/1 -> [IO_CAN2_312_Age]  "<Age>"
  Bus Selector12/2 -> [IO_CAN2_312_cnt]  "<STMM_counterMsg312>"
  Bus Selector12/4 -> Mux12/2  "<STMM_segmentTemp401>"
  IO_CAN2_312_Bus/1 -> Bus Selector12/1
  Bus Selector12/3 -> Mux12/1  "<STMM_segmentTemp400>"
  Bus Selector12/5 -> Mux12/3  "<STMM_segmentTemp402>"
  Bus Selector11/1 -> [IO_CAN2_311_Age]  "<Age>"
  Bus Selector11/2 -> [IO_CAN2_311_cnt]  "<STMM_counterMsg311>"
  Bus Selector11/4 -> Mux11/2  "<STMM_segmentTemp310>"
  Bus Selector11/5 -> Mux11/3  "<STMM_segmentTemp311>"
  Bus Selector11/3 -> Mux11/1  "<STMM_segmentTemp309>"
  IO_CAN2_311_Bus/1 -> Bus Selector11/1
  Bus Selector10/1 -> [IO_CAN2_310_Age]  "<Age>"
  IO_CAN2_310_Bus/1 -> Bus Selector10/1
  Bus Selector10/3 -> Mux10/1  "<STMM_segmentTemp306>"
  Bus Selector10/4 -> Mux10/2  "<STMM_segmentTemp307>"
  Bus Selector10/5 -> Mux10/3  "<STMM_segmentTemp308>"
  Bus Selector10/2 -> [IO_CAN2_310_cnt]  "<STMM_counterMsg310>"
  Bus Selector9/3 -> Mux9/1  "<STMM_segmentTemp303>"
  Bus Selector9/5 -> Mux9/3  "<STMM_segmentTemp305>"
  Bus Selector9/1 -> [IO_CAN2_309_Age]  "<Age>"
  Bus Selector9/4 -> Mux9/2  "<STMM_segmentTemp304>"
  IO_CAN2_309_Bus/1 -> Bus Selector9/1
  Bus Selector9/2 -> [IO_CAN2_309_cnt]  "<STMM_counterMsg309>"
  Bus Selector8/2 -> [IO_CAN2_308_cnt]  "<STMM_counterMsg308>"
  IO_CAN2_308_Bus/1 -> Bus Selector8/1
  Bus Selector8/3 -> Mux8/1  "<STMM_segmentTemp300>"
  Bus Selector8/5 -> Mux8/3  "<STMM_segmentTemp302>"
  Bus Selector8/1 -> [IO_CAN2_308_Age]  "<Age>"
  Bus Selector8/4 -> Mux8/2  "<STMM_segmentTemp301>"
  IO_CAN2_307_Bus/1 -> Bus Selector7/1
  Bus Selector7/5 -> Mux7/3  "<STMM_segmentTemp211>"
  Bus Selector7/4 -> Mux7/2  "<STMM_segmentTemp210>"
  Bus Selector7/1 -> [IO_CAN2_307_Age]  "<Age>"
  Bus Selector7/2 -> [IO_CAN2_307_cnt]  "<STMM_counterMsg307>"
  Bus Selector7/3 -> Mux7/1  "<STMM_segmentTemp209>"
  Bus Selector6/2 -> [IO_CAN2_306_cnt]  "<STMM_counterMsg306>"
  Bus Selector6/3 -> Mux6/1  "<STMM_segmentTemp206>"
  Bus Selector6/5 -> Mux6/3  "<STMM_segmentTemp208>"
  Bus Selector6/4 -> Mux6/2  "<STMM_segmentTemp207>"
  Bus Selector6/1 -> [IO_CAN2_306_Age]  "<Age>"
  IO_CAN2_306_Bus/1 -> Bus Selector6/1
  Bus Selector5/5 -> Mux5/3  "<STMM_segmentTemp205>"
  Bus Selector5/3 -> Mux5/1  "<STMM_segmentTemp203>"
  IO_CAN2_305_Bus/1 -> Bus Selector5/1
  Bus Selector5/1 -> [IO_CAN2_305_Age]  "<Age>"
  Bus Selector5/4 -> Mux5/2  "<STMM_segmentTemp204>"
  Bus Selector5/2 -> [IO_CAN2_305_cnt]  "<STMM_counterMsg305>"
  IO_CAN2_304_Bus/1 -> Bus Selector4/1
  Bus Selector4/4 -> Mux4/2  "<STMM_segmentTemp201>"
  Bus Selector4/3 -> Mux4/1  "<STMM_segmentTemp200>"
  Bus Selector4/5 -> Mux4/3  "<STMM_segmentTemp202>"
  Bus Selector4/2 -> [IO_CAN2_304_cnt]  "<STMM_counterMsg304>"
  Bus Selector4/1 -> [IO_CAN2_304_Age]  "<Age>"
  IO_CAN2_303_Bus/1 -> Bus Selector3/1
  Bus Selector3/4 -> Mux3/2  "<STMM_segmentTemp110>"
  Bus Selector3/3 -> Mux3/1  "<STMM_segmentTemp109>"
  Bus Selector3/1 -> [IO_CAN2_303_Age]  "<Age>"
  Bus Selector3/2 -> [IO_CAN2_303_cnt]  "<STMM_counterMsg303>"
  Bus Selector3/5 -> Mux3/3  "<STMM_segmentTemp111>"
  Bus Selector2/5 -> Mux2/3  "<STMM_segmentTemp108>"
  Bus Selector2/1 -> [IO_CAN2_302_Age]  "<Age>"
  Bus Selector2/2 -> [IO_CAN2_302_cnt]  "<STMM_counterMsg302>"
  Bus Selector2/4 -> Mux2/2  "<STMM_segmentTemp107>"
  Bus Selector2/3 -> Mux2/1  "<STMM_segmentTemp106>"
  IO_CAN2_302_Bus/1 -> Bus Selector2/1
  Bus Selector1/5 -> Mux1/3  "<STMM_segmentTemp105>"
  Bus Selector1/4 -> Mux1/2  "<STMM_segmentTemp104>"
  Bus Selector1/3 -> Mux1/1  "<STMM_segmentTemp103>"
  Bus Selector1/2 -> [IO_CAN2_301_cnt]  "<STMM_counterMsg301>"
  Bus Selector1/1 -> [IO_CAN2_301_Age]  "<Age>"
  IO_CAN2_301_Bus/1 -> Bus Selector1/1
  Bus Selector/5 -> Mux/3  "<STMM_segmentTemp102>"
  Bus Selector/4 -> Mux/2  "<STMM_segmentTemp101>"
  Bus Selector/3 -> Mux/1  "<STMM_segmentTemp100>"
  Bus Selector/2 -> [IO_CAN2_300_cnt]  "<STMM_counterMsg300>"
  Bus Selector/1 -> [IO_CAN2_300_Age]  "<Age>"
  IO_CAN2_300_Bus/1 -> Bus Selector/1
